simulink model "muscleLegs_task2"  (R2025b)
settings: Solver=ode23t  StartTime=0.0  StopTime=t_end  MaxStep=1e-3  RelTol=1e-4
values from neighbouring files (symbols this model uses):
  c = 0.05    [setup_muscleLegs_nm.m]
  CtrlPar = [tau_H_st; phi_K_tgt_st; P_K_st; D_K_st ... (first row only)    [setup_muscleLegs_ctrl.m]
  eref_se = 0.04    [setup_muscleLegs_nm.m]
  FmaxBFSH = 350    [setup_muscleLegs_nm.m]
  FmaxGLU = 4000    [setup_muscleLegs_nm.m]
  FmaxHFL = 2000    [setup_muscleLegs_nm.m]
  FmaxVAS = 5000    [setup_muscleLegs_nm.m]
  g = 9.81    [setup_muscleLegs_model.m]
  G_dtheta_GLU = 5    [setup_muscleLegs_ctrl.m]    (also in sim_muscleLegs_Task2.m = base_G_dtheta_GLU * optim_vals(15); sim_muscleLegs_Task3.m = base_G(2) * optim_vals(15))
  G_theta_GLU = 60    [setup_muscleLegs_ctrl.m]    (also in sim_muscleLegs_Task2.m = base_G_theta_GLU * optim_vals(14); sim_muscleLegs_Task3.m = base_G(1) * optim_vals(14))
  init_stim = 0.01    [setup_muscleLegs_nm.m]
  K = 5    [setup_muscleLegs_nm.m]
  l_HAT = 0.8    [setup_muscleLegs_model.m]
  l_shank = l_leg/2    (= 0.49)    [setup_muscleLegs_model.m]
  l_thigh = l_leg/2    (= 0.49)    [setup_muscleLegs_model.m]
  loptBFSH = 0.12    [setup_muscleLegs_nm.m]
  loptGLU = 0.11    [setup_muscleLegs_nm.m]
  loptHFL = 0.11    [setup_muscleLegs_nm.m]
  loptVAS = 0.08    [setup_muscleLegs_nm.m]
  lslackBFSH = 0.10    (= 0.1)    [setup_muscleLegs_nm.m]
  lslackGLU = 0.13    [setup_muscleLegs_nm.m]
  lslackHFL = 0.10    (= 0.1)    [setup_muscleLegs_nm.m]
  lslackVAS = 0.23    [setup_muscleLegs_nm.m]
  m_HAT = 54    [setup_muscleLegs_model.m]
  m_shank = 4    [setup_muscleLegs_model.m]
  m_thigh = 8    [setup_muscleLegs_model.m]
  N = 12    [cmaes_task1_2_set1.mat]    (also in cmaes_task1_2_set2.mat; cmaes_task2_2_set1.mat = 17; cmaes_task2_2_set2.mat = 17; cmaes_task3_crouch.mat = 17)
  phirefBFSH = 160*pi/180    (= 2.79252680319)    [setup_muscleLegs_nm.m]
  phirefGLU = 60*pi/180    (= 1.0471975512)    [setup_muscleLegs_nm.m]
  phirefHFL = 20*pi/180    (= 0.349065850399)    [setup_muscleLegs_nm.m]
  phirefVAS = 60*pi/180    (= 1.0471975512)    [setup_muscleLegs_nm.m]
  plane_height = 0.1    [setup_muscleLegs_model.m]
  plane_x = 100    [setup_muscleLegs_model.m]
  plane_z = 1    [setup_muscleLegs_model.m]
  r_foot = 0.01    [setup_muscleLegs_model.m]
  rBFSH = 0.04    [setup_muscleLegs_nm.m]
  rGLU = 0.08    [setup_muscleLegs_nm.m]
  rHFL = 0.08    [setup_muscleLegs_nm.m]
  rhoBFSH = 0.7    [setup_muscleLegs_nm.m]
  rhoGLU = 0.5    [setup_muscleLegs_nm.m]
  rhoHFL = 0.5    [setup_muscleLegs_nm.m]
  rhoVAS = 0.6    [setup_muscleLegs_nm.m]
  rVAS = 0.05    [setup_muscleLegs_nm.m]
  tau_act = 0.01    [setup_muscleLegs_nm.m]
  tau_deact = 0.04    [setup_muscleLegs_nm.m]
  theta_tgt = 0.001    [setup_muscleLegs_ctrl.m]    (also in sim_muscleLegs_Task2.m = 0 + (optim_vals(13) - 1) * 0.1; sim_muscleLegs_Task3.m = 0 + (optim_vals(13) - 1) * 0.1)
  vi_Ctrl_st = 1:4    [setup_muscleLegs_ctrl.m]
  vi_Ctrl_sw = 5:12    [setup_muscleLegs_ctrl.m]
  vmaxBFSH = 12    [setup_muscleLegs_nm.m]
  vmaxGLU = 12    [setup_muscleLegs_nm.m]
  vmaxHFL = 12    [setup_muscleLegs_nm.m]
  vmaxVAS = 12    [setup_muscleLegs_nm.m]
  w = 0.56    [setup_muscleLegs_nm.m]
  w_pe = w    (= 0.56)    [setup_muscleLegs_nm.m]
undefined symbols (not defined in the file or in its folder): l1, X, Y, Z
libraries: sm_lib x30, nesl_utility x19, simulink x1
(part 2 of 4)

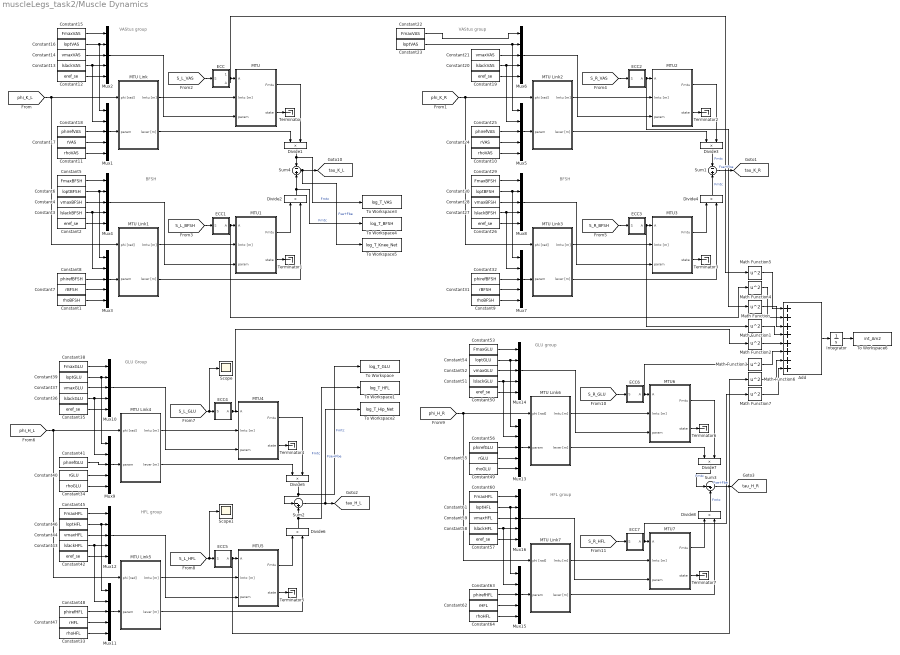
== system muscleLegs_task2/Muscle Dynamics ==
  note: VAStus group
  note: BFSH
  note: VAStus group
  note: BFSH
  note: GLU Group
  note: HFL group
  note: HFL group
  note: GLU group
  Add : Sum  Inputs=++++++++
  Constant1 : Constant  Value=rhoBFSH
  Constant10 : Constant  Value=rhoVAS
  Constant11 : Constant  Value=rhoVAS
  Constant{2,12,19,26,35,42,50,57} (8 alike) : Constant  Value=eref_se
  Constant13 : Constant  Value=lslackVAS
  Constant14 : Constant  Value=vmaxVAS
  Constant15 : Constant  Value=FmaxVAS
  Constant16 : Constant  Value=loptVAS
  Constant17 : Constant  Value=rVAS
  Constant18 : Constant  Value=phirefVAS
  Constant20 : Constant  Value=lslackVAS
  Constant21 : Constant  Value=vmaxVAS
  Constant22 : Constant  Value=FmaxVAS
  Constant23 : Constant  Value=loptVAS
  Constant24 : Constant  Value=rVAS
  Constant25 : Constant  Value=phirefVAS
  Constant27 : Constant  Value=lslackBFSH
  Constant28 : Constant  Value=vmaxBFSH
  Constant29 : Constant  Value=FmaxBFSH
  Constant3 : Constant  Value=lslackBFSH
  Constant30 : Constant  Value=loptBFSH
  Constant31 : Constant  Value=rBFSH
  Constant32 : Constant  Value=phirefBFSH
  Constant33 : Constant  Value=rhoHFL
  Constant34 : Constant  Value=rhoGLU
  Constant36 : Constant  Value=lslackGLU
  Constant37 : Constant  Value=vmaxGLU
  Constant38 : Constant  Value=FmaxGLU
  Constant39 : Constant  Value=loptGLU
  Constant4 : Constant  Value=vmaxBFSH
  Constant40 : Constant  Value=rGLU
  Constant41 : Constant  Value=phirefGLU
  Constant43 : Constant  Value=lslackHFL
  Constant44 : Constant  Value=vmaxHFL
  Constant45 : Constant  Value=FmaxHFL
  Constant46 : Constant  Value=loptHFL
  Constant47 : Constant  Value=rHFL
  Constant48 : Constant  Value=phirefHFL
  Constant49 : Constant  Value=rhoGLU
  Constant5 : Constant  Value=FmaxBFSH
  Constant51 : Constant  Value=lslackGLU
  Constant52 : Constant  Value=vmaxGLU
  Constant53 : Constant  Value=FmaxGLU
  Constant54 : Constant  Value=loptGLU
  Constant55 : Constant  Value=rGLU
  Constant56 : Constant  Value=phirefGLU
  Constant58 : Constant  Value=lslackHFL
  Constant59 : Constant  Value=vmaxHFL
  Constant6 : Constant  Value=loptBFSH
  Constant60 : Constant  Value=FmaxHFL
  Constant61 : Constant  Value=loptHFL
  Constant62 : Constant  Value=rHFL
  Constant63 : Constant  Value=phirefHFL
  Constant64 : Constant  Value=rhoHFL
  Constant7 : Constant  Value=rBFSH
  Constant8 : Constant  Value=phirefBFSH
  Constant9 : Constant  Value=rhoBFSH
  Divide{1..8} (8 alike) : Product
  ECC : Subsystem
  ECC1 : Subsystem
  ECC2 : Subsystem
  ECC3 : Subsystem
  ECC4 : Subsystem
  ECC5 : Subsystem
  ECC6 : Subsystem
  ECC7 : Subsystem
  Integrator : Integrator
  MTU : Subsystem
  MTU Link : Subsystem
  MTU Link1 : Subsystem
  MTU Link2 : Subsystem
  MTU Link3 : Subsystem
  MTU Link4 : Subsystem
  MTU Link5 : Subsystem
  MTU Link6 : Subsystem
  MTU Link7 : Subsystem
  MTU1 : Subsystem
  MTU2 : Subsystem
  MTU3 : Subsystem
  MTU4 : Subsystem
  MTU5 : Subsystem
  MTU6 : Subsystem
  MTU7 : Subsystem
  Math Function{,1..7} (8 alike) : Math  Operator=square
  Mux{1..16} (16 alike) : Mux  Inputs=5
  Scope : Scope
      settings: ActiveDisplayYMinimum=-0.19072734164298966  ActiveDisplayYMaximum=1.1365182783001846
  Scope1 : Scope
      settings: ActiveDisplayYMinimum=-1  ActiveDisplayYMaximum=1  DataLoggingVariableName=ScopeData3
  Sum1 : Sum  Inputs=-+  InputSameDT=on  SaturateOnIntegerOverflow=on  OutDataTypeStr=Inherit: Same as first input
  Sum2 : Sum  Inputs=|-+  InputSameDT=on  SaturateOnIntegerOverflow=on  OutDataTypeStr=Inherit: Same as first input
  Sum3 : Sum  Inputs=|-+  InputSameDT=on  SaturateOnIntegerOverflow=on  OutDataTypeStr=Inherit: Same as first input
  Sum4 : Sum  Inputs=-+  InputSameDT=on  SaturateOnIntegerOverflow=on  OutDataTypeStr=Inherit: Same as first input
  Terminator{,1..7} (8 alike) : Terminator
  To Workspace : ToWorkspace  VariableName=log_T_GLU  SaveFormat=Timeseries  SampleTime=-1
  To Workspace1 : ToWorkspace  VariableName=log_T_HFL  SaveFormat=Timeseries  SampleTime=-1
  To Workspace2 : ToWorkspace  VariableName=log_T_Hip_Net  SaveFormat=Timeseries  SampleTime=-1
  To Workspace3 : ToWorkspace  VariableName=log_T_VAS  SaveFormat=Timeseries  SampleTime=-1
  To Workspace4 : ToWorkspace  VariableName=log_T_BFSH  SaveFormat=Timeseries  SampleTime=-1
  To Workspace5 : ToWorkspace  VariableName=log_T_Knee_Net  SaveFormat=Timeseries  SampleTime=-1
  To Workspace6 : ToWorkspace  VariableName=int_Am2  SaveFormat=Timeseries  SampleTime=-1
  tag scope: tau_H_L=global, tau_H_R=global, tau_K_L=global, tau_K_R=global
  wires:
  Constant11/1 -> Mux1/5
  MTU/2(state) -> Terminator/1
  Constant18/1 -> Mux1/3
  Mux2/1 -> MTU/3(param)
  Constant13/1 -> Mux1/2, Mux2/4
  Constant17/1 -> Mux1/4
  Mux1/1 -> MTU Link/2(param)
  MTU Link/2(lever [m]) -> Divide1/1
  Constant12/1 -> Mux2/5
  MTU/1(Fmtu) -> Divide1/2
  Constant14/1 -> Mux2/3
  Constant16/1 -> Mux1/1, Mux2/2
  MTU Link/1(lmtu [m]) -> MTU/2(lmtc [m])
  Constant15/1 -> Mux2/1
  [S_L_VAS] -> ECC/1(S)
  Divide1/1 -> To Workspace3/1, Sum4/1  "Fmtc"
  Sum4/1 -> To Workspace5/1, [tau_K_L]  "Fse+Fbe"
  [phi_K_L] -> MTU Link/1(phi [rad]), MTU Link1/1(phi [rad])
  Mux3/1 -> MTU Link1/2(param)
  MTU Link1/1(lmtu [m]) -> MTU1/2(lmtc [m])
  [S_L_BFSH] -> ECC1/1(S)
  Constant5/1 -> Mux4/1
  Constant3/1 -> Mux3/2, Mux4/4
  Constant7/1 -> Mux3/4
  Mux4/1 -> MTU1/3(param)
  Constant8/1 -> Mux3/3
  Constant1/1 -> Mux3/5
  MTU1/2(state) -> Terminator1/1
  Constant2/1 -> Mux4/5
  Constant6/1 -> Mux3/1, Mux4/2
  Constant4/1 -> Mux4/3
  MTU1/1(Fmtu) -> Divide2/1
  MTU Link1/2(lever [m]) -> Divide2/2
  Divide2/1 -> To Workspace4/1, Sum4/2  "Fmtc"
  Divide4/1 -> Sum1/2  "Fmtc"
  [S_R_BFSH] -> ECC3/1(S)
  [phi_K_R] -> MTU Link2/1(phi [rad]), MTU Link3/1(phi [rad])
  Mux5/1 -> MTU Link2/2(param)
  MTU Link2/2(lever [m]) -> Divide3/1
  Constant22/1 -> Mux6/1
  Constant20/1 -> Mux5/2, Mux6/4
  Constant24/1 -> Mux5/4
  Constant25/1 -> Mux5/3
  Constant10/1 -> Mux5/5
  Divide3/1 -> Sum1/1  "Fmtc"
  Constant28/1 -> Mux8/3
  Constant9/1 -> Mux7/5
  Constant30/1 -> Mux7/1, Mux8/2
  MTU3/2(state) -> Terminator3/1
  Constant32/1 -> Mux7/3
  MTU2/2(state) -> Terminator2/1
  Mux8/1 -> MTU3/3(param)
  MTU Link3/2(lever [m]) -> Divide4/2
  MTU Link3/1(lmtu [m]) -> MTU3/2(lmtc [m])
  Constant27/1 -> Mux7/2, Mux8/4
  Constant29/1 -> Mux8/1
  Mux7/1 -> MTU Link3/2(param)
  MTU Link2/1(lmtu [m]) -> MTU2/2(lmtc [m])
  MTU2/1(Fmtu) -> Divide3/2
  Constant19/1 -> Mux6/5
  Mux6/1 -> MTU2/3(param)
  MTU3/1(Fmtu) -> Divide4/1
  Constant26/1 -> Mux8/5
  Constant31/1 -> Mux7/4
  Constant23/1 -> Mux5/1, Mux6/2
  Sum1/1 -> [tau_K_R]  "Fse+Fbe"
  Constant21/1 -> Mux6/3
  ECC1/1(A) -> Math Function4/1, MTU1/1(A)
  [S_R_VAS] -> ECC2/1(S)
  ECC2/1(A) -> Math Function/1, MTU2/1(A)
  ECC3/1(A) -> Math Function1/1, MTU3/1(A)
  MTU4/2(state) -> Terminator4/1
  Constant40/1 -> Mux9/4
  Divide5/1 -> To Workspace/1, Sum2/1  "Fmtc"
  Mux10/1 -> MTU4/3(param)
  MTU Link4/1(lmtu [m]) -> MTU4/2(lmtc [m])
  Constant48/1 -> Mux11/3
  MTU4/1(Fmtu) -> Divide5/2
  MTU5/2(state) -> Terminator5/1
  MTU Link5/2(lever [m]) -> Divide6/2
  Constant36/1 -> Mux9/2, Mux10/4
  ECC5/1(A) -> Math Function6/1, MTU5/1(A)
  Constant41/1 -> Mux9/3
  Constant45/1 -> Mux12/1
  Constant44/1 -> Mux12/3
  MTU Link5/1(lmtu [m]) -> MTU5/2(lmtc [m])
  Divide6/1 -> To Workspace1/1, Sum2/2  "Fmtc"
  MTU5/1(Fmtu) -> Divide6/1
  Constant39/1 -> Mux9/1, Mux10/2
  Constant38/1 -> Mux10/1
  Constant34/1 -> Mux9/5
  [phi_H_L] -> MTU Link4/1(phi [rad]), MTU Link5/1(phi [rad])
  Mux12/1 -> MTU5/3(param)
  Constant43/1 -> Mux11/2, Mux12/4
  [S_L_GLU] -> Scope/1, ECC4/1(S)
  Sum2/1 -> To Workspace2/1, [tau_H_L]  "Fse+Fbe"
  Mux11/1 -> MTU Link5/2(param)
  ECC4/1(A) -> Math Function2/1, MTU4/1(A)
  MTU Link4/2(lever [m]) -> Divide5/1
  Constant46/1 -> Mux11/1, Mux12/2
  Constant35/1 -> Mux10/5
  Constant37/1 -> Mux10/3
  Constant42/1 -> Mux12/5
  Mux9/1 -> MTU Link4/2(param)
  Constant33/1 -> Mux11/5
  Constant47/1 -> Mux11/4
  Constant53/1 -> Mux14/1
  Mux13/1 -> MTU Link6/2(param)
  MTU Link6/1(lmtu [m]) -> MTU6/2(lmtc [m])
  Constant60/1 -> Mux16/1
  Mux16/1 -> MTU7/3(param)
  Mux14/1 -> MTU6/3(param)
  Divide8/1 -> Sum3/2  "Fmtc"
  MTU6/2(state) -> Terminator6/1
  Constant64/1 -> Mux15/5
  Constant59/1 -> Mux16/3
  Constant61/1 -> Mux15/1, Mux16/2
  MTU6/1(Fmtu) -> Divide7/2
  ECC6/1(A) -> Math Function3/1, MTU6/1(A)
  [phi_H_R] -> MTU Link6/1(phi [rad]), MTU Link7/1(phi [rad])
  Constant49/1 -> Mux13/5
  Constant55/1 -> Mux13/4
  Mux15/1 -> MTU Link7/2(param)
  Divide7/1 -> Sum3/1  "Fmtc"
  Constant56/1 -> Mux13/3
  Constant62/1 -> Mux15/4
  Constant54/1 -> Mux13/1, Mux14/2
  [S_R_GLU] -> ECC6/1(S)
  Constant63/1 -> Mux15/3
  Constant52/1 -> Mux14/3
  MTU Link6/2(lever [m]) -> Divide7/1
  ECC7/1(A) -> Math Function7/1, MTU7/1(A)
  Constant57/1 -> Mux16/5
  MTU7/2(state) -> Terminator7/1
  MTU Link7/1(lmtu [m]) -> MTU7/2(lmtc [m])
  Constant50/1 -> Mux14/5
  Constant51/1 -> Mux13/2, Mux14/4
  Sum3/1 -> [tau_H_R]  "Fse+Fbe"
  MTU Link7/2(lever [m]) -> Divide8/2
  MTU7/1(Fmtu) -> Divide8/1
  [S_R_HFL] -> ECC7/1(S)
  Constant58/1 -> Mux15/2, Mux16/4
  [S_L_HFL] -> Scope1/1, ECC5/1(S)
  ECC/2(A) -> Math Function5/1, MTU/1(A)
  Math Function5/1 -> Add/1
  Math Function4/1 -> Add/2
  Math Function/1 -> Add/3
  Math Function1/1 -> Add/4
  Math Function2/1 -> Add/5
  Math Function3/1 -> Add/6
  Math Function6/1 -> Add/7
  Math Function7/1 -> Add/8
  Add/1 -> Integrator/1
  Integrator/1 -> To Workspace6/1

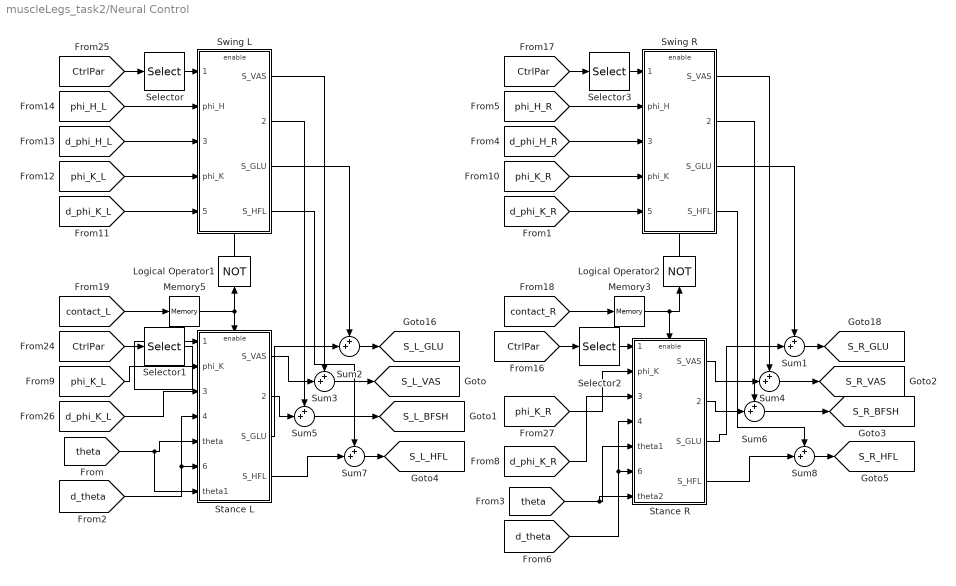
== system muscleLegs_task2/Neural Control ==
  Logical Operator1 : Logic  Operator=NOT  AllPortsSameDT=off  OutDataTypeStr=boolean
  Logical Operator2 : Logic  Operator=NOT  AllPortsSameDT=off  OutDataTypeStr=boolean
  Memory3 : Memory
  Memory5 : Memory  InitialCondition=1
  Selector : Selector  InputPortWidth=length(CtrlPar)  IndexOptions=Index vector (dialog)  Indices=vi_Ctrl_sw  OutputSizes=1
  Selector1 : Selector  InputPortWidth=length(CtrlPar)  IndexOptions=Index vector (dialog)  Indices=vi_Ctrl_st  OutputSizes=1
  Selector2 : Selector  InputPortWidth=length(CtrlPar)  IndexOptions=Index vector (dialog)  Indices=vi_Ctrl_st  OutputSizes=1
  Selector3 : Selector  InputPortWidth=length(CtrlPar)  IndexOptions=Index vector (dialog)  Indices=vi_Ctrl_sw  OutputSizes=1
  Stance L : Subsystem
  Stance R : Subsystem
  Sum{1..8} (8 alike) : Sum  Inputs=++|
  Swing L : Subsystem
  Swing R : Subsystem
  tag scope: S_L_BFSH=global, S_L_GLU=global, S_L_HFL=global, S_L_VAS=global, S_R_BFSH=global, S_R_GLU=global, S_R_HFL=global, S_R_VAS=global
  wires:
  [contact_R] -> Memory3/1
  [phi_K_R] -> Swing R/4(phi_K)
  Sum2/1 -> [S_L_GLU]
  Logical Operator1/1 -> Swing L/Enable
  Memory5/1 -> Logical Operator1/1, Stance L/Enable
  Selector1/1 -> Stance L/1(CtrlPar)
  [CtrlPar] -> Selector2/1
  Memory3/1 -> Logical Operator2/1, Stance R/Enable
  [phi_H_L] -> Swing L/2(phi_H)
  [d_phi_K_L] -> Stance L/3(d_phi_K)
  Logical Operator2/1 -> Swing R/Enable
  [d_phi_K_R] -> Stance R/3(d_phi_K)
  [d_phi_H_L] -> Swing L/3(d_phi_H)
  Sum1/1 -> [S_R_GLU]
  [d_phi_K_L] -> Swing L/5(d_phi_K)
  [d_phi_H_R] -> Swing R/3(d_phi_H)
  [d_phi_K_R] -> Swing R/5(d_phi_K)
  [phi_H_R] -> Swing R/2(phi_H)
  [CtrlPar] -> Selector/1
  [CtrlPar] -> Selector1/1
  Selector3/1 -> Swing R/1(CtrlPar)
  [phi_K_R] -> Stance R/2(phi_K)
  Selector/1 -> Swing L/1(CtrlPar)
  Selector2/1 -> Stance R/1(CtrlPar)
  [CtrlPar] -> Selector3/1
  [phi_K_L] -> Stance L/2(phi_K)
  [phi_K_L] -> Swing L/4(phi_K)
  [contact_L] -> Memory5/1
  Swing L/1(S_VAS) -> Sum3/1
  Swing L/2(S_BFSH) -> Sum5/1
  Sum3/1 -> [S_L_VAS]
  Stance L/1(S_VAS) -> Sum3/2
  Stance L/2(S_BFSH) -> Sum5/2
  Sum5/1 -> [S_L_BFSH]
  Stance R/2(S_BFSH) -> Sum6/2
  Stance R/1(S_VAS) -> Sum4/2
  Sum4/1 -> [S_R_VAS]
  Sum6/1 -> [S_R_BFSH]
  Swing R/2(S_BFSH) -> Sum6/1
  Swing R/1(S_VAS) -> Sum4/1
  Swing L/3(S_GLU) -> Sum2/1
  Stance L/3(S_GLU) -> Sum2/2
  Sum7/1 -> [S_L_HFL]
  Swing L/4(S_HFL) -> Sum7/1
  Stance L/4(S_HFL) -> Sum7/2
  Swing R/3(S_GLU) -> Sum1/1
  Stance R/3(S_GLU) -> Sum1/2
  Sum8/1 -> [S_R_HFL]
  Swing R/4(S_HFL) -> Sum8/1
  Stance R/4(S_HFL) -> Sum8/2
  [theta] -> Stance L/7(theta1), Stance L/5(theta)
  [d_theta] -> Stance L/6(d_theta1), Stance L/4(d_theta)
  [theta] -> Stance R/7(theta2), Stance R/5(theta1)
  [d_theta] -> Stance R/6(d_theta2), Stance R/4(d_theta1)

== system muscleLegs_task2/Muscle Dynamics/ECC ==
  S : Inport
  Constant : Constant  Value=tau_act
  Constant1 : Constant  Value=tau_deact
  Divide : Product  Inputs=*/
  Integrator : Integrator  InitialCondition=init_stim
  Sum : Sum  Inputs=+-|
  Switch : Switch  Criteria=u2 > Threshold  SaturateOnIntegerOverflow=off  InputSameDT=off
  Out1 : Outport
  A : Outport  Port=2  VectorParamsAs1DForOutWhenUnconnected=off
  wires:
  S/1 -> Sum/1
  Integrator/1 -> A/1, Sum/2  "A"
  Divide/1 -> Integrator/1  "dA"
  Sum/1 -> Divide/1, Switch/2
  Switch/1 -> Divide/2
  Constant/1 -> Switch/1
  Constant1/1 -> Switch/3

== system muscleLegs_task2/Muscle Dynamics/ECC1 ==
  S : Inport
  Constant : Constant  Value=tau_act
  Constant1 : Constant  Value=tau_deact
  Divide : Product  Inputs=*/
  Integrator : Integrator  InitialCondition=init_stim
  Sum : Sum  Inputs=+-|
  Switch : Switch  Criteria=u2 > Threshold  SaturateOnIntegerOverflow=off  InputSameDT=off
  A : Outport  VectorParamsAs1DForOutWhenUnconnected=off
  wires:
  S/1 -> Sum/1
  Integrator/1 -> A/1, Sum/2  "A"
  Divide/1 -> Integrator/1  "dA"
  Sum/1 -> Divide/1, Switch/2
  Switch/1 -> Divide/2
  Constant/1 -> Switch/1
  Constant1/1 -> Switch/3

== system muscleLegs_task2/Muscle Dynamics/ECC2 ==
  S : Inport
  Constant : Constant  Value=tau_act
  Constant1 : Constant  Value=tau_deact
  Divide : Product  Inputs=*/
  Integrator : Integrator  InitialCondition=init_stim
  Sum : Sum  Inputs=+-|
  Switch : Switch  Criteria=u2 > Threshold  SaturateOnIntegerOverflow=off  InputSameDT=off
  A : Outport  VectorParamsAs1DForOutWhenUnconnected=off
  wires:
  S/1 -> Sum/1
  Integrator/1 -> A/1, Sum/2  "A"
  Divide/1 -> Integrator/1  "dA"
  Sum/1 -> Divide/1, Switch/2
  Switch/1 -> Divide/2
  Constant/1 -> Switch/1
  Constant1/1 -> Switch/3

== system muscleLegs_task2/Muscle Dynamics/ECC3 ==
  S : Inport
  Constant : Constant  Value=tau_act
  Constant1 : Constant  Value=tau_deact
  Divide : Product  Inputs=*/
  Integrator : Integrator  InitialCondition=init_stim
  Sum : Sum  Inputs=+-|
  Switch : Switch  Criteria=u2 > Threshold  SaturateOnIntegerOverflow=off  InputSameDT=off
  A : Outport  VectorParamsAs1DForOutWhenUnconnected=off
  wires:
  S/1 -> Sum/1
  Integrator/1 -> A/1, Sum/2  "A"
  Divide/1 -> Integrator/1  "dA"
  Sum/1 -> Divide/1, Switch/2
  Switch/1 -> Divide/2
  Constant/1 -> Switch/1
  Constant1/1 -> Switch/3

== system muscleLegs_task2/Muscle Dynamics/ECC4 ==
  S : Inport
  Constant : Constant  Value=tau_act
  Constant1 : Constant  Value=tau_deact
  Divide : Product  Inputs=*/
  Integrator : Integrator  InitialCondition=init_stim
  Sum : Sum  Inputs=+-|
  Switch : Switch  Criteria=u2 > Threshold  SaturateOnIntegerOverflow=off  InputSameDT=off
  A : Outport  VectorParamsAs1DForOutWhenUnconnected=off
  wires:
  S/1 -> Sum/1
  Integrator/1 -> A/1, Sum/2  "A"
  Divide/1 -> Integrator/1  "dA"
  Sum/1 -> Divide/1, Switch/2
  Switch/1 -> Divide/2
  Constant/1 -> Switch/1
  Constant1/1 -> Switch/3

== system muscleLegs_task2/Muscle Dynamics/ECC5 ==
  S : Inport
  Constant : Constant  Value=tau_act
  Constant1 : Constant  Value=tau_deact
  Divide : Product  Inputs=*/
  Integrator : Integrator  InitialCondition=init_stim
  Sum : Sum  Inputs=+-|
  Switch : Switch  Criteria=u2 > Threshold  SaturateOnIntegerOverflow=off  InputSameDT=off
  A : Outport  VectorParamsAs1DForOutWhenUnconnected=off
  wires:
  S/1 -> Sum/1
  Integrator/1 -> A/1, Sum/2  "A"
  Divide/1 -> Integrator/1  "dA"
  Sum/1 -> Divide/1, Switch/2
  Switch/1 -> Divide/2
  Constant/1 -> Switch/1
  Constant1/1 -> Switch/3

== system muscleLegs_task2/Muscle Dynamics/ECC6 ==
  S : Inport
  Constant : Constant  Value=tau_act
  Constant1 : Constant  Value=tau_deact
  Divide : Product  Inputs=*/
  Integrator : Integrator  InitialCondition=init_stim
  Sum : Sum  Inputs=+-|
  Switch : Switch  Criteria=u2 > Threshold  SaturateOnIntegerOverflow=off  InputSameDT=off
  A : Outport  VectorParamsAs1DForOutWhenUnconnected=off
  wires:
  S/1 -> Sum/1
  Integrator/1 -> A/1, Sum/2  "A"
  Divide/1 -> Integrator/1  "dA"
  Sum/1 -> Divide/1, Switch/2
  Switch/1 -> Divide/2
  Constant/1 -> Switch/1
  Constant1/1 -> Switch/3

== system muscleLegs_task2/Muscle Dynamics/ECC7 ==
  S : Inport
  Constant : Constant  Value=tau_act
  Constant1 : Constant  Value=tau_deact
  Divide : Product  Inputs=*/
  Integrator : Integrator  InitialCondition=init_stim
  Sum : Sum  Inputs=+-|
  Switch : Switch  Criteria=u2 > Threshold  SaturateOnIntegerOverflow=off  InputSameDT=off
  A : Outport  VectorParamsAs1DForOutWhenUnconnected=off
  wires:
  S/1 -> Sum/1
  Integrator/1 -> A/1, Sum/2  "A"
  Divide/1 -> Integrator/1  "dA"
  Sum/1 -> Divide/1, Switch/2
  Switch/1 -> Divide/2
  Constant/1 -> Switch/1
  Constant1/1 -> Switch/3

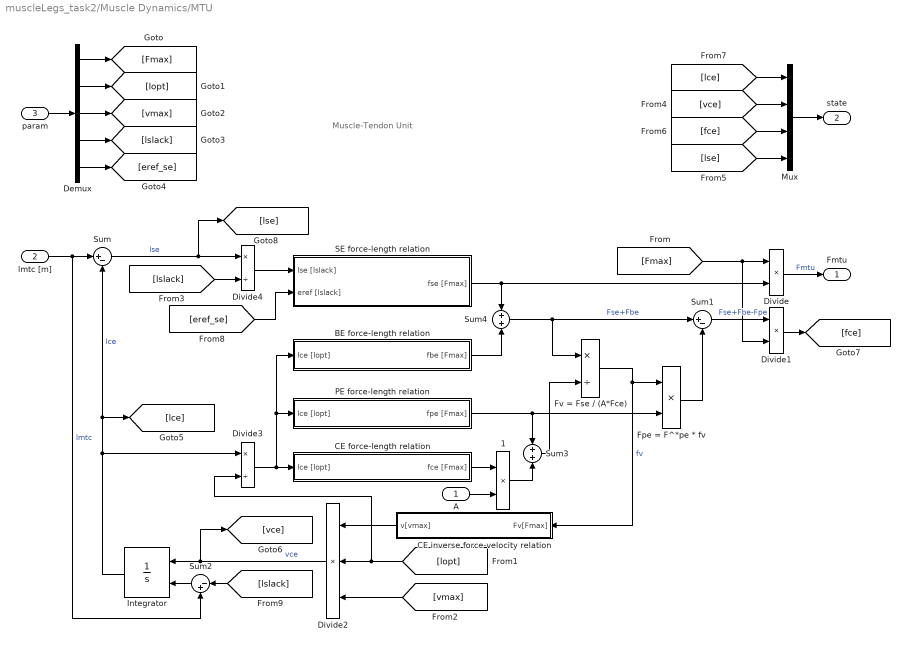
== system muscleLegs_task2/Muscle Dynamics/MTU ==
  note: Muscle-Tendon Unit
  A : Inport
  lmtc [m] : Inport  Port=2
  param : Inport  Port=3
  1 : Product  Inputs=**  InputSameDT=on  SaturateOnIntegerOverflow=on  OutDataTypeStr=Inherit: Same as first input
  BE force-length relation : Subsystem
  CE force-length relation : Subsystem
  CE inverse force-velocity relation : Subsystem
  Demux : Demux  Outputs=5
  Divide : Product
  Divide1 : Product
  Divide2 : Product  Inputs=3
  Divide3 : Product  Inputs=*/
  Divide4 : Product  Inputs=*/
  "Fpe = F^*pe * fv " : Product  InputSameDT=on  SaturateOnIntegerOverflow=on  OutDataTypeStr=Inherit: Same as first input
  Fv = Fse / (A*Fce) : Product  Inputs=*/  InputSameDT=on  SaturateOnIntegerOverflow=on  OutDataTypeStr=Inherit: Same as first input
  Integrator : Integrator  InitialConditionSource=external  LowerSaturationLimit=0.05
  Mux : Mux
  PE force-length relation : Subsystem
  SE force-length relation : Subsystem
  Sum : Sum  Inputs=|+-  InputSameDT=on  SaturateOnIntegerOverflow=on  OutDataTypeStr=Inherit: Same as first input
  Sum1 : Sum  Inputs=|+-  InputSameDT=on  SaturateOnIntegerOverflow=on  OutDataTypeStr=Inherit: Same as first input
  Sum2 : Sum  Inputs=|-+  InputSameDT=on  SaturateOnIntegerOverflow=on  OutDataTypeStr=Inherit: Same as first input
  Sum3 : Sum  InputSameDT=on  SaturateOnIntegerOverflow=on  OutDataTypeStr=Inherit: Same as first input
  Sum4 : Sum  InputSameDT=on  SaturateOnIntegerOverflow=on  OutDataTypeStr=Inherit: Same as first input
  Fmtu : Outport  InitialOutput=0  VectorParamsAs1DForOutWhenUnconnected=off
  state : Outport  Port=2  InitialOutput=0  VectorParamsAs1DForOutWhenUnconnected=off
  wires:
  Integrator/1 -> Divide3/1, [lce], Sum/2  "lce"
  Divide3/1 -> CE force-length relation/1(lce [lopt]), PE force-length relation/1(lce [lopt]), BE force-length relation/1(lce [lopt])
  Fv = Fse / (A*Fce)/1 -> CE inverse force-velocity relation/1(Fv[Fmax]), "Fpe = F^*pe * fv "/1  "fv"
  Divide2/1 -> [vce], Integrator/1  "vce"
  lmtc [m]/1 -> Sum/1, Sum2/2  "lmtc"
  Divide/1 -> Fmtu/1  "Fmtu"
  Divide4/1 -> SE force-length relation/1(lse [lslack])
  SE force-length relation/1(fse [Fmax]) -> Sum4/1, Divide/2
  Sum2/1 -> Integrator/2
  [lslack] -> Sum2/1
  CE force-length relation/1(fce [Fmax]) -> 1/1
  PE force-length relation/1(fpe [Fmax]) -> "Fpe = F^*pe * fv "/2, Sum3/1
  1/1 -> Sum3/2
  BE force-length relation/1(fbe [Fmax]) -> Sum4/2
  Sum3/1 -> Fv = Fse / (A*Fce)/2
  CE inverse force-velocity relation/1(v[vmax]) -> Divide2/1
  A/1 -> 1/2
  Sum4/1 -> Sum1/1, Fv = Fse / (A*Fce)/1  "Fse+Fbe"
  "Fpe = F^*pe * fv "/1 -> Sum1/2
  Sum1/1 -> Divide1/1  "Fse+Fbe-Fpe"
  Divide1/1 -> [fce]
  Sum/1 -> [lse], Divide4/1  "lse"
  [lopt] -> Divide2/2, Divide3/2
  [vmax] -> Divide2/3
  [lslack] -> Divide4/2
  param/1 -> Demux/1
  Demux/1 -> [Fmax]
  Demux/2 -> [lopt]
  Demux/4 -> [lslack]
  Demux/3 -> [vmax]
  Demux/5 -> [eref_se]
  [Fmax] -> Divide1/2, Divide/1
  Mux/1 -> state/1
  [lce] -> Mux/1
  [vce] -> Mux/2
  [fce] -> Mux/3
  [lse] -> Mux/4
  [eref_se] -> SE force-length relation/2(eref [lslack])

== system muscleLegs_task2/Muscle Dynamics/MTU Link ==
  note: check sign:
      | ++: larger phi -> longer mtu
      | +-: larger phi -> shorter mtu
  note: Muscle Attachment
  phi [rad] : Inport
  param : Inport  Port=2
  Demux : Demux  Outputs=5
  Product : Product  Inputs=3  RndMeth=Zero
  Sum1 : Sum  Inputs=|++
  Sum2 : Sum  Inputs=|+-
  Sum5 : Sum  Inputs=|++
  lmtu [m] : Outport  VectorParamsAs1DForOutWhenUnconnected=off
  lever [m] : Outport  Port=2  VectorParamsAs1DForOutWhenUnconnected=off
  wires:
  Sum1/1 -> Sum5/1
  Sum5/1 -> lmtu [m]/1
  phi [rad]/1 -> Sum2/1
  Demux/3 -> Sum2/2  "phiref"
  Sum2/1 -> Product/1
  Demux/4 -> lever [m]/1, Product/2  "r"
  Product/1 -> Sum5/2
  Demux/1 -> Sum1/1  "lopt"
  Demux/2 -> Sum1/2  "lslack"
  Demux/5 -> Product/3  "rho"
  param/1 -> Demux/1

== system muscleLegs_task2/Muscle Dynamics/MTU Link1 ==
  note: check sign:
      | ++: larger phi -> longer mtu
      | +-: larger phi -> shorter mtu
  note: Muscle Attachment
  phi [rad] : Inport
  param : Inport  Port=2
  Demux : Demux  Outputs=5
  Product : Product  Inputs=3  RndMeth=Zero
  Sum1 : Sum  Inputs=|++
  Sum2 : Sum  Inputs=|+-
  Sum5 : Sum  Inputs=|+-
  lmtu [m] : Outport  VectorParamsAs1DForOutWhenUnconnected=off
  lever [m] : Outport  Port=2  VectorParamsAs1DForOutWhenUnconnected=off
  wires:
  Sum1/1 -> Sum5/1
  Sum5/1 -> lmtu [m]/1
  phi [rad]/1 -> Sum2/1
  Demux/3 -> Sum2/2  "phiref"
  Sum2/1 -> Product/1
  Demux/4 -> lever [m]/1, Product/2  "r"
  Product/1 -> Sum5/2
  Demux/1 -> Sum1/1  "lopt"
  Demux/2 -> Sum1/2  "lslack"
  Demux/5 -> Product/3  "rho"
  param/1 -> Demux/1

== system muscleLegs_task2/Muscle Dynamics/MTU Link2 ==
  note: check sign:
      | ++: larger phi -> longer mtu
      | +-: larger phi -> shorter mtu
  note: Muscle Attachment
  phi [rad] : Inport
  param : Inport  Port=2
  Demux : Demux  Outputs=5
  Product : Product  Inputs=3  RndMeth=Zero
  Sum1 : Sum  Inputs=|++
  Sum2 : Sum  Inputs=|+-
  Sum5 : Sum  Inputs=|++
  lmtu [m] : Outport  VectorParamsAs1DForOutWhenUnconnected=off
  lever [m] : Outport  Port=2  VectorParamsAs1DForOutWhenUnconnected=off
  wires:
  Sum1/1 -> Sum5/1
  Sum5/1 -> lmtu [m]/1
  phi [rad]/1 -> Sum2/1
  Demux/3 -> Sum2/2  "phiref"
  Sum2/1 -> Product/1
  Demux/4 -> lever [m]/1, Product/2  "r"
  Product/1 -> Sum5/2
  Demux/1 -> Sum1/1  "lopt"
  Demux/2 -> Sum1/2  "lslack"
  Demux/5 -> Product/3  "rho"
  param/1 -> Demux/1

== system muscleLegs_task2/Muscle Dynamics/MTU Link3 ==
  note: check sign:
      | ++: larger phi -> longer mtu
      | +-: larger phi -> shorter mtu
  note: Muscle Attachment
  phi [rad] : Inport
  param : Inport  Port=2
  Demux : Demux  Outputs=5
  Product : Product  Inputs=3  RndMeth=Zero
  Sum1 : Sum  Inputs=|++
  Sum2 : Sum  Inputs=|+-
  Sum5 : Sum  Inputs=|+-
  lmtu [m] : Outport  VectorParamsAs1DForOutWhenUnconnected=off
  lever [m] : Outport  Port=2  VectorParamsAs1DForOutWhenUnconnected=off
  wires:
  Sum1/1 -> Sum5/1
  Sum5/1 -> lmtu [m]/1
  phi [rad]/1 -> Sum2/1
  Demux/3 -> Sum2/2  "phiref"
  Sum2/1 -> Product/1
  Demux/4 -> lever [m]/1, Product/2  "r"
  Product/1 -> Sum5/2
  Demux/1 -> Sum1/1  "lopt"
  Demux/2 -> Sum1/2  "lslack"
  Demux/5 -> Product/3  "rho"
  param/1 -> Demux/1

== system muscleLegs_task2/Muscle Dynamics/MTU Link4 ==
  note: check sign:
      | ++: larger phi -> longer mtu
      | +-: larger phi -> shorter mtu
  note: Muscle Attachment
  phi [rad] : Inport
  param : Inport  Port=2
  Demux : Demux  Outputs=5
  Product : Product  Inputs=3  RndMeth=Zero
  Sum1 : Sum  Inputs=|++
  Sum2 : Sum  Inputs=|+-
  Sum5 : Sum  Inputs=|++
  lmtu [m] : Outport  VectorParamsAs1DForOutWhenUnconnected=off
  lever [m] : Outport  Port=2  VectorParamsAs1DForOutWhenUnconnected=off
  wires:
  Sum1/1 -> Sum5/1
  Sum5/1 -> lmtu [m]/1
  phi [rad]/1 -> Sum2/1
  Demux/3 -> Sum2/2  "phiref"
  Sum2/1 -> Product/1
  Demux/4 -> lever [m]/1, Product/2  "r"
  Product/1 -> Sum5/2
  Demux/1 -> Sum1/1  "lopt"
  Demux/2 -> Sum1/2  "lslack"
  Demux/5 -> Product/3  "rho"
  param/1 -> Demux/1

== system muscleLegs_task2/Muscle Dynamics/MTU Link5 ==
  note: check sign:
      | ++: larger phi -> longer mtu
      | +-: larger phi -> shorter mtu
  note: Muscle Attachment
  phi [rad] : Inport
  param : Inport  Port=2
  Demux : Demux  Outputs=5
  Product : Product  Inputs=3  RndMeth=Zero
  Sum1 : Sum  Inputs=|++
  Sum2 : Sum  Inputs=|+-
  Sum5 : Sum  Inputs=|+-
  lmtu [m] : Outport  VectorParamsAs1DForOutWhenUnconnected=off
  lever [m] : Outport  Port=2  VectorParamsAs1DForOutWhenUnconnected=off
  wires:
  Sum1/1 -> Sum5/1
  Sum5/1 -> lmtu [m]/1
  phi [rad]/1 -> Sum2/1
  Demux/3 -> Sum2/2  "phiref"
  Sum2/1 -> Product/1
  Demux/4 -> lever [m]/1, Product/2  "r"
  Product/1 -> Sum5/2
  Demux/1 -> Sum1/1  "lopt"
  Demux/2 -> Sum1/2  "lslack"
  Demux/5 -> Product/3  "rho"
  param/1 -> Demux/1

== system muscleLegs_task2/Muscle Dynamics/MTU Link6 ==
  note: check sign:
      | ++: larger phi -> longer mtu
      | +-: larger phi -> shorter mtu
  note: Muscle Attachment
  phi [rad] : Inport
  param : Inport  Port=2
  Demux : Demux  Outputs=5
  Product : Product  Inputs=3  RndMeth=Zero
  Sum1 : Sum  Inputs=|++
  Sum2 : Sum  Inputs=|+-
  Sum5 : Sum  Inputs=|++
  lmtu [m] : Outport  VectorParamsAs1DForOutWhenUnconnected=off
  lever [m] : Outport  Port=2  VectorParamsAs1DForOutWhenUnconnected=off
  wires:
  Sum1/1 -> Sum5/1
  Sum5/1 -> lmtu [m]/1
  phi [rad]/1 -> Sum2/1
  Demux/3 -> Sum2/2  "phiref"
  Sum2/1 -> Product/1
  Demux/4 -> lever [m]/1, Product/2  "r"
  Product/1 -> Sum5/2
  Demux/1 -> Sum1/1  "lopt"
  Demux/2 -> Sum1/2  "lslack"
  Demux/5 -> Product/3  "rho"
  param/1 -> Demux/1

== system muscleLegs_task2/Muscle Dynamics/MTU Link7 ==
  note: check sign:
      | ++: larger phi -> longer mtu
      | +-: larger phi -> shorter mtu
  note: Muscle Attachment
  phi [rad] : Inport
  param : Inport  Port=2
  Demux : Demux  Outputs=5
  Product : Product  Inputs=3  RndMeth=Zero
  Sum1 : Sum  Inputs=|++
  Sum2 : Sum  Inputs=|+-
  Sum5 : Sum  Inputs=|+-
  lmtu [m] : Outport  VectorParamsAs1DForOutWhenUnconnected=off
  lever [m] : Outport  Port=2  VectorParamsAs1DForOutWhenUnconnected=off
  wires:
  Sum1/1 -> Sum5/1
  Sum5/1 -> lmtu [m]/1
  phi [rad]/1 -> Sum2/1
  Demux/3 -> Sum2/2  "phiref"
  Sum2/1 -> Product/1
  Demux/4 -> lever [m]/1, Product/2  "r"
  Product/1 -> Sum5/2
  Demux/1 -> Sum1/1  "lopt"
  Demux/2 -> Sum1/2  "lslack"
  Demux/5 -> Product/3  "rho"
  param/1 -> Demux/1

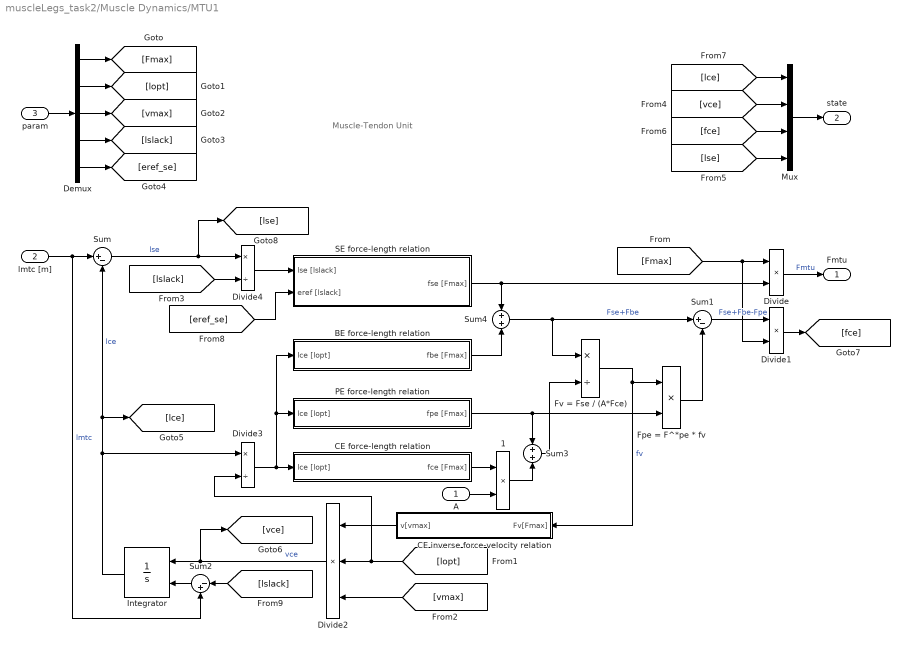
== system muscleLegs_task2/Muscle Dynamics/MTU1 ==
  note: Muscle-Tendon Unit
  A : Inport
  lmtc [m] : Inport  Port=2
  param : Inport  Port=3
  1 : Product  Inputs=**  InputSameDT=on  SaturateOnIntegerOverflow=on  OutDataTypeStr=Inherit: Same as first input
  BE force-length relation : Subsystem
  CE force-length relation : Subsystem
  CE inverse force-velocity relation : Subsystem
  Demux : Demux  Outputs=5
  Divide : Product
  Divide1 : Product
  Divide2 : Product  Inputs=3
  Divide3 : Product  Inputs=*/
  Divide4 : Product  Inputs=*/
  "Fpe = F^*pe * fv " : Product  InputSameDT=on  SaturateOnIntegerOverflow=on  OutDataTypeStr=Inherit: Same as first input
  Fv = Fse / (A*Fce) : Product  Inputs=*/  InputSameDT=on  SaturateOnIntegerOverflow=on  OutDataTypeStr=Inherit: Same as first input
  Integrator : Integrator  InitialConditionSource=external  LowerSaturationLimit=0.05
  Mux : Mux
  PE force-length relation : Subsystem
  SE force-length relation : Subsystem
  Sum : Sum  Inputs=|+-  InputSameDT=on  SaturateOnIntegerOverflow=on  OutDataTypeStr=Inherit: Same as first input
  Sum1 : Sum  Inputs=|+-  InputSameDT=on  SaturateOnIntegerOverflow=on  OutDataTypeStr=Inherit: Same as first input
  Sum2 : Sum  Inputs=|-+  InputSameDT=on  SaturateOnIntegerOverflow=on  OutDataTypeStr=Inherit: Same as first input
  Sum3 : Sum  InputSameDT=on  SaturateOnIntegerOverflow=on  OutDataTypeStr=Inherit: Same as first input
  Sum4 : Sum  InputSameDT=on  SaturateOnIntegerOverflow=on  OutDataTypeStr=Inherit: Same as first input
  Fmtu : Outport  InitialOutput=0  VectorParamsAs1DForOutWhenUnconnected=off
  state : Outport  Port=2  InitialOutput=0  VectorParamsAs1DForOutWhenUnconnected=off
  wires:
  Integrator/1 -> Divide3/1, [lce], Sum/2  "lce"
  Divide3/1 -> CE force-length relation/1(lce [lopt]), PE force-length relation/1(lce [lopt]), BE force-length relation/1(lce [lopt])
  Fv = Fse / (A*Fce)/1 -> CE inverse force-velocity relation/1(Fv[Fmax]), "Fpe = F^*pe * fv "/1  "fv"
  Divide2/1 -> [vce], Integrator/1  "vce"
  lmtc [m]/1 -> Sum/1, Sum2/2  "lmtc"
  Divide/1 -> Fmtu/1  "Fmtu"
  Divide4/1 -> SE force-length relation/1(lse [lslack])
  SE force-length relation/1(fse [Fmax]) -> Sum4/1, Divide/2
  Sum2/1 -> Integrator/2
  [lslack] -> Sum2/1
  CE force-length relation/1(fce [Fmax]) -> 1/1
  PE force-length relation/1(fpe [Fmax]) -> "Fpe = F^*pe * fv "/2, Sum3/1
  1/1 -> Sum3/2
  BE force-length relation/1(fbe [Fmax]) -> Sum4/2
  Sum3/1 -> Fv = Fse / (A*Fce)/2
  CE inverse force-velocity relation/1(v[vmax]) -> Divide2/1
  A/1 -> 1/2
  Sum4/1 -> Sum1/1, Fv = Fse / (A*Fce)/1  "Fse+Fbe"
  "Fpe = F^*pe * fv "/1 -> Sum1/2
  Sum1/1 -> Divide1/1  "Fse+Fbe-Fpe"
  Divide1/1 -> [fce]
  Sum/1 -> [lse], Divide4/1  "lse"
  [lopt] -> Divide2/2, Divide3/2
  [vmax] -> Divide2/3
  [lslack] -> Divide4/2
  param/1 -> Demux/1
  Demux/1 -> [Fmax]
  Demux/2 -> [lopt]
  Demux/4 -> [lslack]
  Demux/3 -> [vmax]
  Demux/5 -> [eref_se]
  [Fmax] -> Divide1/2, Divide/1
  Mux/1 -> state/1
  [lce] -> Mux/1
  [vce] -> Mux/2
  [fce] -> Mux/3
  [lse] -> Mux/4
  [eref_se] -> SE force-length relation/2(eref [lslack])

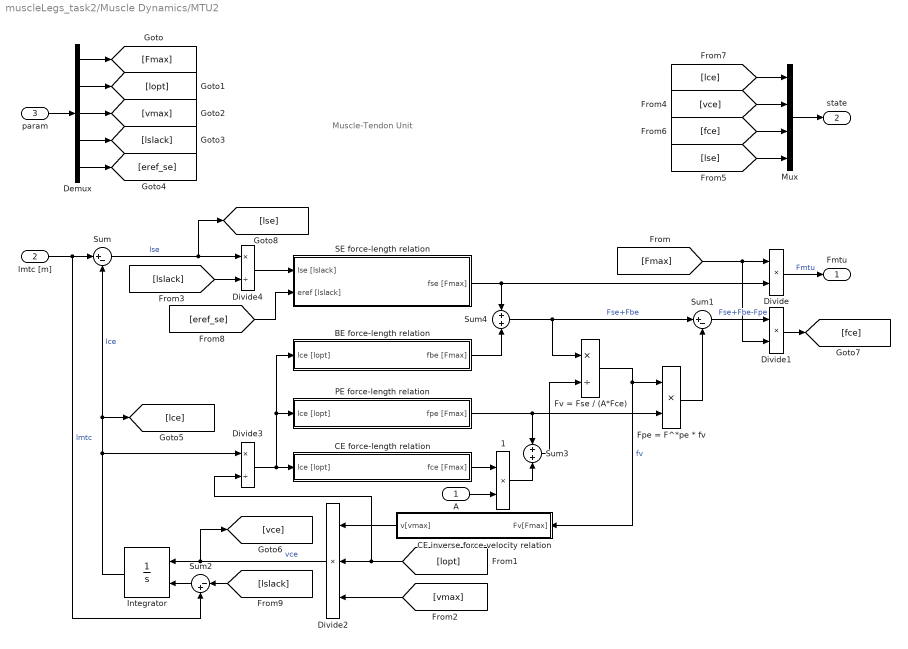
== system muscleLegs_task2/Muscle Dynamics/MTU2 ==
  note: Muscle-Tendon Unit
  A : Inport
  lmtc [m] : Inport  Port=2
  param : Inport  Port=3
  1 : Product  Inputs=**  InputSameDT=on  SaturateOnIntegerOverflow=on  OutDataTypeStr=Inherit: Same as first input
  BE force-length relation : Subsystem
  CE force-length relation : Subsystem
  CE inverse force-velocity relation : Subsystem
  Demux : Demux  Outputs=5
  Divide : Product
  Divide1 : Product
  Divide2 : Product  Inputs=3
  Divide3 : Product  Inputs=*/
  Divide4 : Product  Inputs=*/
  "Fpe = F^*pe * fv " : Product  InputSameDT=on  SaturateOnIntegerOverflow=on  OutDataTypeStr=Inherit: Same as first input
  Fv = Fse / (A*Fce) : Product  Inputs=*/  InputSameDT=on  SaturateOnIntegerOverflow=on  OutDataTypeStr=Inherit: Same as first input
  Integrator : Integrator  InitialConditionSource=external  LowerSaturationLimit=0.05
  Mux : Mux
  PE force-length relation : Subsystem
  SE force-length relation : Subsystem
  Sum : Sum  Inputs=|+-  InputSameDT=on  SaturateOnIntegerOverflow=on  OutDataTypeStr=Inherit: Same as first input
  Sum1 : Sum  Inputs=|+-  InputSameDT=on  SaturateOnIntegerOverflow=on  OutDataTypeStr=Inherit: Same as first input
  Sum2 : Sum  Inputs=|-+  InputSameDT=on  SaturateOnIntegerOverflow=on  OutDataTypeStr=Inherit: Same as first input
  Sum3 : Sum  InputSameDT=on  SaturateOnIntegerOverflow=on  OutDataTypeStr=Inherit: Same as first input
  Sum4 : Sum  InputSameDT=on  SaturateOnIntegerOverflow=on  OutDataTypeStr=Inherit: Same as first input
  Fmtu : Outport  InitialOutput=0  VectorParamsAs1DForOutWhenUnconnected=off
  state : Outport  Port=2  InitialOutput=0  VectorParamsAs1DForOutWhenUnconnected=off
  wires:
  Integrator/1 -> Divide3/1, [lce], Sum/2  "lce"
  Divide3/1 -> CE force-length relation/1(lce [lopt]), PE force-length relation/1(lce [lopt]), BE force-length relation/1(lce [lopt])
  Fv = Fse / (A*Fce)/1 -> CE inverse force-velocity relation/1(Fv[Fmax]), "Fpe = F^*pe * fv "/1  "fv"
  Divide2/1 -> [vce], Integrator/1  "vce"
  lmtc [m]/1 -> Sum/1, Sum2/2  "lmtc"
  Divide/1 -> Fmtu/1  "Fmtu"
  Divide4/1 -> SE force-length relation/1(lse [lslack])
  SE force-length relation/1(fse [Fmax]) -> Sum4/1, Divide/2
  Sum2/1 -> Integrator/2
  [lslack] -> Sum2/1
  CE force-length relation/1(fce [Fmax]) -> 1/1
  PE force-length relation/1(fpe [Fmax]) -> "Fpe = F^*pe * fv "/2, Sum3/1
  1/1 -> Sum3/2
  BE force-length relation/1(fbe [Fmax]) -> Sum4/2
  Sum3/1 -> Fv = Fse / (A*Fce)/2
  CE inverse force-velocity relation/1(v[vmax]) -> Divide2/1
  A/1 -> 1/2
  Sum4/1 -> Sum1/1, Fv = Fse / (A*Fce)/1  "Fse+Fbe"
  "Fpe = F^*pe * fv "/1 -> Sum1/2
  Sum1/1 -> Divide1/1  "Fse+Fbe-Fpe"
  Divide1/1 -> [fce]
  Sum/1 -> [lse], Divide4/1  "lse"
  [lopt] -> Divide2/2, Divide3/2
  [vmax] -> Divide2/3
  [lslack] -> Divide4/2
  param/1 -> Demux/1
  Demux/1 -> [Fmax]
  Demux/2 -> [lopt]
  Demux/4 -> [lslack]
  Demux/3 -> [vmax]
  Demux/5 -> [eref_se]
  [Fmax] -> Divide1/2, Divide/1
  Mux/1 -> state/1
  [lce] -> Mux/1
  [vce] -> Mux/2
  [fce] -> Mux/3
  [lse] -> Mux/4
  [eref_se] -> SE force-length relation/2(eref [lslack])

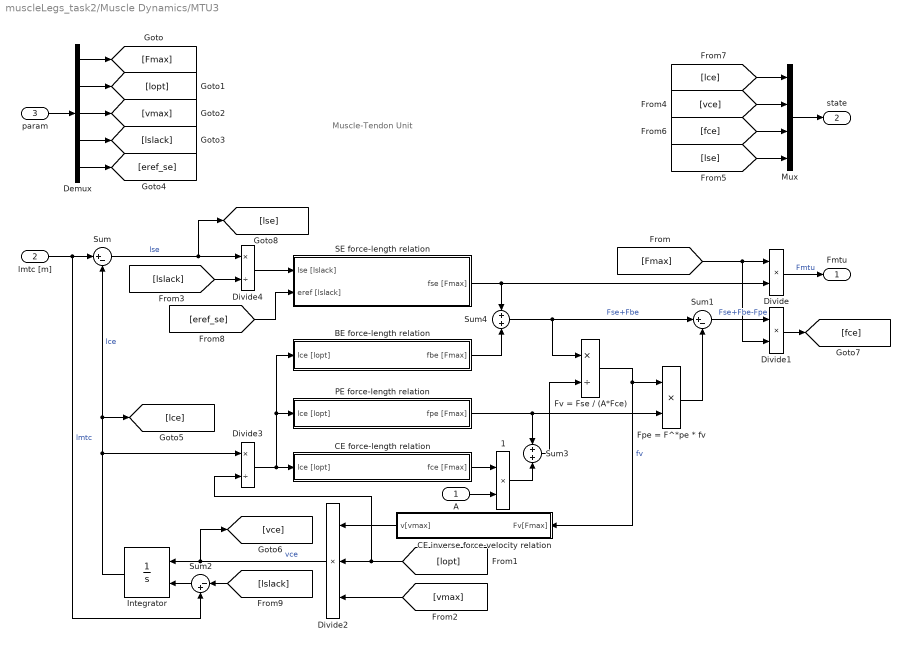
== system muscleLegs_task2/Muscle Dynamics/MTU3 ==
  note: Muscle-Tendon Unit
  A : Inport
  lmtc [m] : Inport  Port=2
  param : Inport  Port=3
  1 : Product  Inputs=**  InputSameDT=on  SaturateOnIntegerOverflow=on  OutDataTypeStr=Inherit: Same as first input
  BE force-length relation : Subsystem
  CE force-length relation : Subsystem
  CE inverse force-velocity relation : Subsystem
  Demux : Demux  Outputs=5
  Divide : Product
  Divide1 : Product
  Divide2 : Product  Inputs=3
  Divide3 : Product  Inputs=*/
  Divide4 : Product  Inputs=*/
  "Fpe = F^*pe * fv " : Product  InputSameDT=on  SaturateOnIntegerOverflow=on  OutDataTypeStr=Inherit: Same as first input
  Fv = Fse / (A*Fce) : Product  Inputs=*/  InputSameDT=on  SaturateOnIntegerOverflow=on  OutDataTypeStr=Inherit: Same as first input
  Integrator : Integrator  InitialConditionSource=external  LowerSaturationLimit=0.05
  Mux : Mux
  PE force-length relation : Subsystem
  SE force-length relation : Subsystem
  Sum : Sum  Inputs=|+-  InputSameDT=on  SaturateOnIntegerOverflow=on  OutDataTypeStr=Inherit: Same as first input
  Sum1 : Sum  Inputs=|+-  InputSameDT=on  SaturateOnIntegerOverflow=on  OutDataTypeStr=Inherit: Same as first input
  Sum2 : Sum  Inputs=|-+  InputSameDT=on  SaturateOnIntegerOverflow=on  OutDataTypeStr=Inherit: Same as first input
  Sum3 : Sum  InputSameDT=on  SaturateOnIntegerOverflow=on  OutDataTypeStr=Inherit: Same as first input
  Sum4 : Sum  InputSameDT=on  SaturateOnIntegerOverflow=on  OutDataTypeStr=Inherit: Same as first input
  Fmtu : Outport  InitialOutput=0  VectorParamsAs1DForOutWhenUnconnected=off
  state : Outport  Port=2  InitialOutput=0  VectorParamsAs1DForOutWhenUnconnected=off
  wires:
  Integrator/1 -> Divide3/1, [lce], Sum/2  "lce"
  Divide3/1 -> CE force-length relation/1(lce [lopt]), PE force-length relation/1(lce [lopt]), BE force-length relation/1(lce [lopt])
  Fv = Fse / (A*Fce)/1 -> CE inverse force-velocity relation/1(Fv[Fmax]), "Fpe = F^*pe * fv "/1  "fv"
  Divide2/1 -> [vce], Integrator/1  "vce"
  lmtc [m]/1 -> Sum/1, Sum2/2  "lmtc"
  Divide/1 -> Fmtu/1  "Fmtu"
  Divide4/1 -> SE force-length relation/1(lse [lslack])
  SE force-length relation/1(fse [Fmax]) -> Sum4/1, Divide/2
  Sum2/1 -> Integrator/2
  [lslack] -> Sum2/1
  CE force-length relation/1(fce [Fmax]) -> 1/1
  PE force-length relation/1(fpe [Fmax]) -> "Fpe = F^*pe * fv "/2, Sum3/1
  1/1 -> Sum3/2
  BE force-length relation/1(fbe [Fmax]) -> Sum4/2
  Sum3/1 -> Fv = Fse / (A*Fce)/2
  CE inverse force-velocity relation/1(v[vmax]) -> Divide2/1
  A/1 -> 1/2
  Sum4/1 -> Sum1/1, Fv = Fse / (A*Fce)/1  "Fse+Fbe"
  "Fpe = F^*pe * fv "/1 -> Sum1/2
  Sum1/1 -> Divide1/1  "Fse+Fbe-Fpe"
  Divide1/1 -> [fce]
  Sum/1 -> [lse], Divide4/1  "lse"
  [lopt] -> Divide2/2, Divide3/2
  [vmax] -> Divide2/3
  [lslack] -> Divide4/2
  param/1 -> Demux/1
  Demux/1 -> [Fmax]
  Demux/2 -> [lopt]
  Demux/4 -> [lslack]
  Demux/3 -> [vmax]
  Demux/5 -> [eref_se]
  [Fmax] -> Divide1/2, Divide/1
  Mux/1 -> state/1
  [lce] -> Mux/1
  [vce] -> Mux/2
  [fce] -> Mux/3
  [lse] -> Mux/4
  [eref_se] -> SE force-length relation/2(eref [lslack])

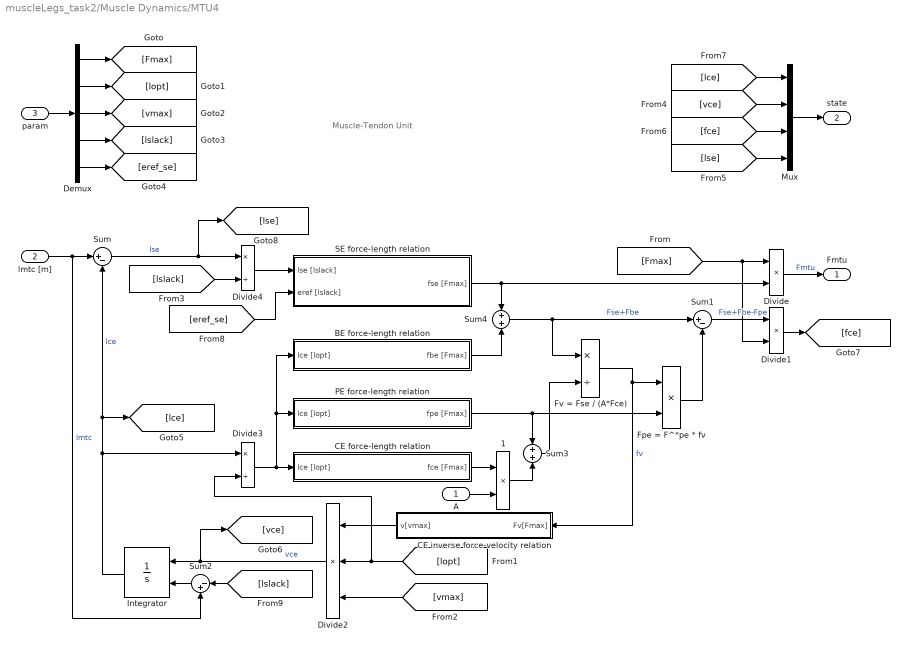
== system muscleLegs_task2/Muscle Dynamics/MTU4 ==
  note: Muscle-Tendon Unit
  A : Inport
  lmtc [m] : Inport  Port=2
  param : Inport  Port=3
  1 : Product  Inputs=**  InputSameDT=on  SaturateOnIntegerOverflow=on  OutDataTypeStr=Inherit: Same as first input
  BE force-length relation : Subsystem
  CE force-length relation : Subsystem
  CE inverse force-velocity relation : Subsystem
  Demux : Demux  Outputs=5
  Divide : Product
  Divide1 : Product
  Divide2 : Product  Inputs=3
  Divide3 : Product  Inputs=*/
  Divide4 : Product  Inputs=*/
  "Fpe = F^*pe * fv " : Product  InputSameDT=on  SaturateOnIntegerOverflow=on  OutDataTypeStr=Inherit: Same as first input
  Fv = Fse / (A*Fce) : Product  Inputs=*/  InputSameDT=on  SaturateOnIntegerOverflow=on  OutDataTypeStr=Inherit: Same as first input
  Integrator : Integrator  InitialConditionSource=external  LowerSaturationLimit=0.05
  Mux : Mux
  PE force-length relation : Subsystem
  SE force-length relation : Subsystem
  Sum : Sum  Inputs=|+-  InputSameDT=on  SaturateOnIntegerOverflow=on  OutDataTypeStr=Inherit: Same as first input
  Sum1 : Sum  Inputs=|+-  InputSameDT=on  SaturateOnIntegerOverflow=on  OutDataTypeStr=Inherit: Same as first input
  Sum2 : Sum  Inputs=|-+  InputSameDT=on  SaturateOnIntegerOverflow=on  OutDataTypeStr=Inherit: Same as first input
  Sum3 : Sum  InputSameDT=on  SaturateOnIntegerOverflow=on  OutDataTypeStr=Inherit: Same as first input
  Sum4 : Sum  InputSameDT=on  SaturateOnIntegerOverflow=on  OutDataTypeStr=Inherit: Same as first input
  Fmtu : Outport  InitialOutput=0  VectorParamsAs1DForOutWhenUnconnected=off
  state : Outport  Port=2  InitialOutput=0  VectorParamsAs1DForOutWhenUnconnected=off
  wires:
  Integrator/1 -> Divide3/1, [lce], Sum/2  "lce"
  Divide3/1 -> CE force-length relation/1(lce [lopt]), PE force-length relation/1(lce [lopt]), BE force-length relation/1(lce [lopt])
  Fv = Fse / (A*Fce)/1 -> CE inverse force-velocity relation/1(Fv[Fmax]), "Fpe = F^*pe * fv "/1  "fv"
  Divide2/1 -> [vce], Integrator/1  "vce"
  lmtc [m]/1 -> Sum/1, Sum2/2  "lmtc"
  Divide/1 -> Fmtu/1  "Fmtu"
  Divide4/1 -> SE force-length relation/1(lse [lslack])
  SE force-length relation/1(fse [Fmax]) -> Sum4/1, Divide/2
  Sum2/1 -> Integrator/2
  [lslack] -> Sum2/1
  CE force-length relation/1(fce [Fmax]) -> 1/1
  PE force-length relation/1(fpe [Fmax]) -> "Fpe = F^*pe * fv "/2, Sum3/1
  1/1 -> Sum3/2
  BE force-length relation/1(fbe [Fmax]) -> Sum4/2
  Sum3/1 -> Fv = Fse / (A*Fce)/2
  CE inverse force-velocity relation/1(v[vmax]) -> Divide2/1
  A/1 -> 1/2
  Sum4/1 -> Sum1/1, Fv = Fse / (A*Fce)/1  "Fse+Fbe"
  "Fpe = F^*pe * fv "/1 -> Sum1/2
  Sum1/1 -> Divide1/1  "Fse+Fbe-Fpe"
  Divide1/1 -> [fce]
  Sum/1 -> [lse], Divide4/1  "lse"
  [lopt] -> Divide2/2, Divide3/2
  [vmax] -> Divide2/3
  [lslack] -> Divide4/2
  param/1 -> Demux/1
  Demux/1 -> [Fmax]
  Demux/2 -> [lopt]
  Demux/4 -> [lslack]
  Demux/3 -> [vmax]
  Demux/5 -> [eref_se]
  [Fmax] -> Divide1/2, Divide/1
  Mux/1 -> state/1
  [lce] -> Mux/1
  [vce] -> Mux/2
  [fce] -> Mux/3
  [lse] -> Mux/4
  [eref_se] -> SE force-length relation/2(eref [lslack])

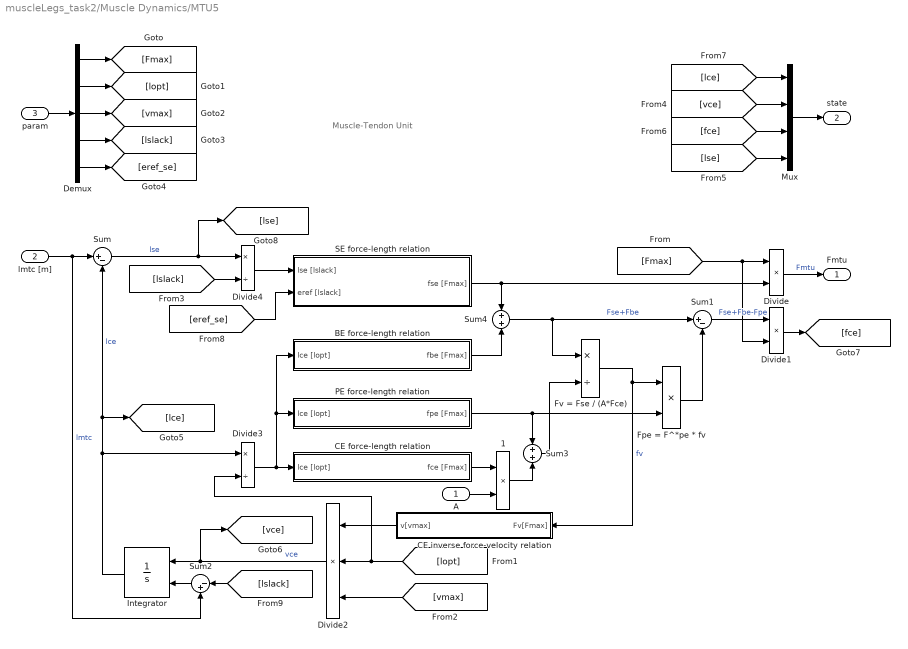
== system muscleLegs_task2/Muscle Dynamics/MTU5 ==
  note: Muscle-Tendon Unit
  A : Inport
  lmtc [m] : Inport  Port=2
  param : Inport  Port=3
  1 : Product  Inputs=**  InputSameDT=on  SaturateOnIntegerOverflow=on  OutDataTypeStr=Inherit: Same as first input
  BE force-length relation : Subsystem
  CE force-length relation : Subsystem
  CE inverse force-velocity relation : Subsystem
  Demux : Demux  Outputs=5
  Divide : Product
  Divide1 : Product
  Divide2 : Product  Inputs=3
  Divide3 : Product  Inputs=*/
  Divide4 : Product  Inputs=*/
  "Fpe = F^*pe * fv " : Product  InputSameDT=on  SaturateOnIntegerOverflow=on  OutDataTypeStr=Inherit: Same as first input
  Fv = Fse / (A*Fce) : Product  Inputs=*/  InputSameDT=on  SaturateOnIntegerOverflow=on  OutDataTypeStr=Inherit: Same as first input
  Integrator : Integrator  InitialConditionSource=external  LowerSaturationLimit=0.05
  Mux : Mux
  PE force-length relation : Subsystem
  SE force-length relation : Subsystem
  Sum : Sum  Inputs=|+-  InputSameDT=on  SaturateOnIntegerOverflow=on  OutDataTypeStr=Inherit: Same as first input
  Sum1 : Sum  Inputs=|+-  InputSameDT=on  SaturateOnIntegerOverflow=on  OutDataTypeStr=Inherit: Same as first input
  Sum2 : Sum  Inputs=|-+  InputSameDT=on  SaturateOnIntegerOverflow=on  OutDataTypeStr=Inherit: Same as first input
  Sum3 : Sum  InputSameDT=on  SaturateOnIntegerOverflow=on  OutDataTypeStr=Inherit: Same as first input
  Sum4 : Sum  InputSameDT=on  SaturateOnIntegerOverflow=on  OutDataTypeStr=Inherit: Same as first input
  Fmtu : Outport  InitialOutput=0  VectorParamsAs1DForOutWhenUnconnected=off
  state : Outport  Port=2  InitialOutput=0  VectorParamsAs1DForOutWhenUnconnected=off
  wires:
  Integrator/1 -> Divide3/1, [lce], Sum/2  "lce"
  Divide3/1 -> CE force-length relation/1(lce [lopt]), PE force-length relation/1(lce [lopt]), BE force-length relation/1(lce [lopt])
  Fv = Fse / (A*Fce)/1 -> CE inverse force-velocity relation/1(Fv[Fmax]), "Fpe = F^*pe * fv "/1  "fv"
  Divide2/1 -> [vce], Integrator/1  "vce"
  lmtc [m]/1 -> Sum/1, Sum2/2  "lmtc"
  Divide/1 -> Fmtu/1  "Fmtu"
  Divide4/1 -> SE force-length relation/1(lse [lslack])
  SE force-length relation/1(fse [Fmax]) -> Sum4/1, Divide/2
  Sum2/1 -> Integrator/2
  [lslack] -> Sum2/1
  CE force-length relation/1(fce [Fmax]) -> 1/1
  PE force-length relation/1(fpe [Fmax]) -> "Fpe = F^*pe * fv "/2, Sum3/1
  1/1 -> Sum3/2
  BE force-length relation/1(fbe [Fmax]) -> Sum4/2
  Sum3/1 -> Fv = Fse / (A*Fce)/2
  CE inverse force-velocity relation/1(v[vmax]) -> Divide2/1
  A/1 -> 1/2
  Sum4/1 -> Sum1/1, Fv = Fse / (A*Fce)/1  "Fse+Fbe"
  "Fpe = F^*pe * fv "/1 -> Sum1/2
  Sum1/1 -> Divide1/1  "Fse+Fbe-Fpe"
  Divide1/1 -> [fce]
  Sum/1 -> [lse], Divide4/1  "lse"
  [lopt] -> Divide2/2, Divide3/2
  [vmax] -> Divide2/3
  [lslack] -> Divide4/2
  param/1 -> Demux/1
  Demux/1 -> [Fmax]
  Demux/2 -> [lopt]
  Demux/4 -> [lslack]
  Demux/3 -> [vmax]
  Demux/5 -> [eref_se]
  [Fmax] -> Divide1/2, Divide/1
  Mux/1 -> state/1
  [lce] -> Mux/1
  [vce] -> Mux/2
  [fce] -> Mux/3
  [lse] -> Mux/4
  [eref_se] -> SE force-length relation/2(eref [lslack])

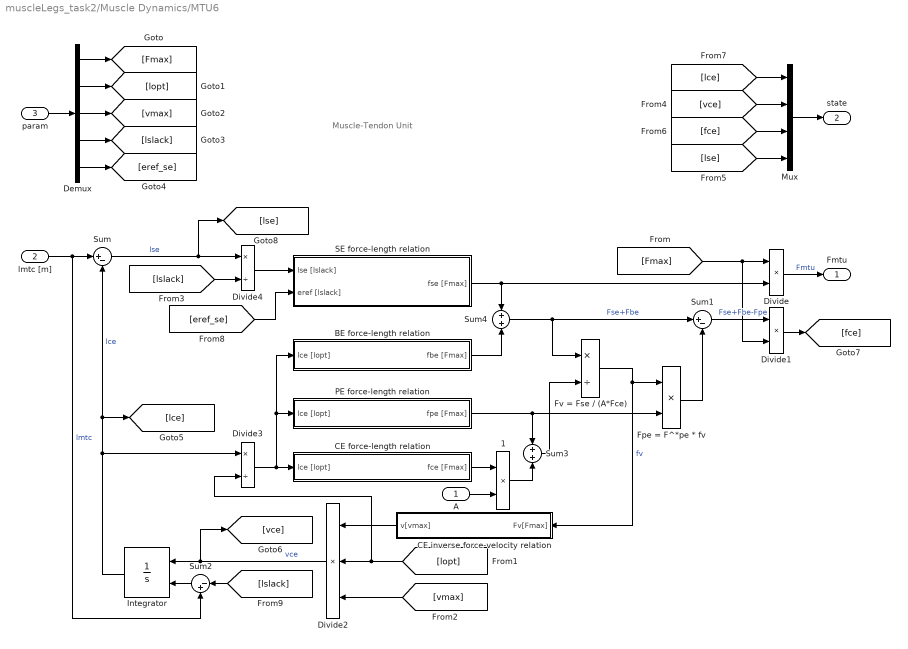
== system muscleLegs_task2/Muscle Dynamics/MTU6 ==
  note: Muscle-Tendon Unit
  A : Inport
  lmtc [m] : Inport  Port=2
  param : Inport  Port=3
  1 : Product  Inputs=**  InputSameDT=on  SaturateOnIntegerOverflow=on  OutDataTypeStr=Inherit: Same as first input
  BE force-length relation : Subsystem
  CE force-length relation : Subsystem
  CE inverse force-velocity relation : Subsystem
  Demux : Demux  Outputs=5
  Divide : Product
  Divide1 : Product
  Divide2 : Product  Inputs=3
  Divide3 : Product  Inputs=*/
  Divide4 : Product  Inputs=*/
  "Fpe = F^*pe * fv " : Product  InputSameDT=on  SaturateOnIntegerOverflow=on  OutDataTypeStr=Inherit: Same as first input
  Fv = Fse / (A*Fce) : Product  Inputs=*/  InputSameDT=on  SaturateOnIntegerOverflow=on  OutDataTypeStr=Inherit: Same as first input
  Integrator : Integrator  InitialConditionSource=external  LowerSaturationLimit=0.05
  Mux : Mux
  PE force-length relation : Subsystem
  SE force-length relation : Subsystem
  Sum : Sum  Inputs=|+-  InputSameDT=on  SaturateOnIntegerOverflow=on  OutDataTypeStr=Inherit: Same as first input
  Sum1 : Sum  Inputs=|+-  InputSameDT=on  SaturateOnIntegerOverflow=on  OutDataTypeStr=Inherit: Same as first input
  Sum2 : Sum  Inputs=|-+  InputSameDT=on  SaturateOnIntegerOverflow=on  OutDataTypeStr=Inherit: Same as first input
  Sum3 : Sum  InputSameDT=on  SaturateOnIntegerOverflow=on  OutDataTypeStr=Inherit: Same as first input
  Sum4 : Sum  InputSameDT=on  SaturateOnIntegerOverflow=on  OutDataTypeStr=Inherit: Same as first input
  Fmtu : Outport  InitialOutput=0  VectorParamsAs1DForOutWhenUnconnected=off
  state : Outport  Port=2  InitialOutput=0  VectorParamsAs1DForOutWhenUnconnected=off
  wires:
  Integrator/1 -> Divide3/1, [lce], Sum/2  "lce"
  Divide3/1 -> CE force-length relation/1(lce [lopt]), PE force-length relation/1(lce [lopt]), BE force-length relation/1(lce [lopt])
  Fv = Fse / (A*Fce)/1 -> CE inverse force-velocity relation/1(Fv[Fmax]), "Fpe = F^*pe * fv "/1  "fv"
  Divide2/1 -> [vce], Integrator/1  "vce"
  lmtc [m]/1 -> Sum/1, Sum2/2  "lmtc"
  Divide/1 -> Fmtu/1  "Fmtu"
  Divide4/1 -> SE force-length relation/1(lse [lslack])
  SE force-length relation/1(fse [Fmax]) -> Sum4/1, Divide/2
  Sum2/1 -> Integrator/2
  [lslack] -> Sum2/1
  CE force-length relation/1(fce [Fmax]) -> 1/1
  PE force-length relation/1(fpe [Fmax]) -> "Fpe = F^*pe * fv "/2, Sum3/1
  1/1 -> Sum3/2
  BE force-length relation/1(fbe [Fmax]) -> Sum4/2
  Sum3/1 -> Fv = Fse / (A*Fce)/2
  CE inverse force-velocity relation/1(v[vmax]) -> Divide2/1
  A/1 -> 1/2
  Sum4/1 -> Sum1/1, Fv = Fse / (A*Fce)/1  "Fse+Fbe"
  "Fpe = F^*pe * fv "/1 -> Sum1/2
  Sum1/1 -> Divide1/1  "Fse+Fbe-Fpe"
  Divide1/1 -> [fce]
  Sum/1 -> [lse], Divide4/1  "lse"
  [lopt] -> Divide2/2, Divide3/2
  [vmax] -> Divide2/3
  [lslack] -> Divide4/2
  param/1 -> Demux/1
  Demux/1 -> [Fmax]
  Demux/2 -> [lopt]
  Demux/4 -> [lslack]
  Demux/3 -> [vmax]
  Demux/5 -> [eref_se]
  [Fmax] -> Divide1/2, Divide/1
  Mux/1 -> state/1
  [lce] -> Mux/1
  [vce] -> Mux/2
  [fce] -> Mux/3
  [lse] -> Mux/4
  [eref_se] -> SE force-length relation/2(eref [lslack])
